simulink model "Model"  (R2015a)
settings: Solver=ode45  StartTime=0.0  StopTime=10.0  RelTol=1e-3
values from neighbouring files (symbols this model uses):
  A = [0          1          0           0 ... (first row only)    [ss_model.m]
  B = [0; 1; 0; 0]    [ss_model.m]
  C = [1 0 0 0 ... (first row only)    [ss_model.m]
  ctrl = 500/s    [ss_model.m]
  D = zeros(2,1)    [ss_model.m]
  Ke = -1.0000e+05    (= -100000)    [ss_model.m]    (also in synthesis.m)
  L = 0.0220    (= 0.022)    [ss_model.m]    (also in synthesis.m)
  R = 1.3    [ss_model.m]    (also in synthesis.m)
settings Model: CovModelRefEnable=off  Creator=gsavaia  LastModifiedBy=user
settings DataIOCC: SaveFormat=Dataset
settings HardwareCC: ProdBitPerPointer=64  ProdLargestAtomicFloat=Float  ProdIntDivRoundTo=Zero  ProdEndianess=LittleEndian  ProdHWDeviceType=Specified
settings GRTTargetCC: GeneratePreprocessorConditionals=Use local settings

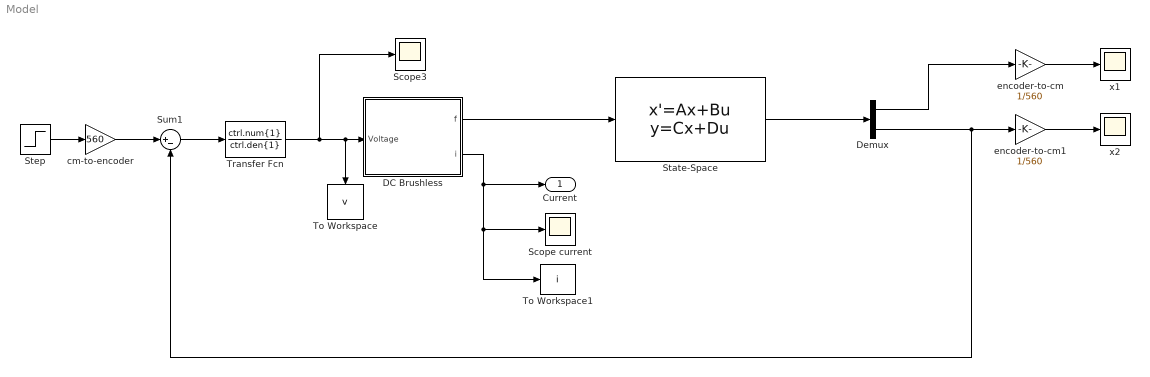
== system Model ==
  DC Brushless : Subsystem
  Demux : Demux  Outputs=2
  Scope current : Scope
      settings: YMin=-0.525  YMax=4.725
  Scope3 : Scope
      settings: TimeRange=2.475095785440614  YMin=3885000.000000001  YMax=8411666.666666668  SaveName=ScopeData4
  State-Space : StateSpace  A=A  B=B  C=C  D=D  X0=0
  Step : Step  SampleTime=0
  Sum1 : Sum  Inputs=|+-
  To Workspace : ToWorkspace  VariableName=v  SaveFormat=Timeseries  SampleTime=-1
  To Workspace1 : ToWorkspace  VariableName=i  SaveFormat=Timeseries  SampleTime=-1
  Transfer Fcn : TransferFcn  Numerator=ctrl.num{1}  Denominator=ctrl.den{1}
  cm-to-encoder : Gain  Gain=560
  encoder-to-cm : Gain  Gain=1/560
  encoder-to-cm1 : Gain  Gain=1/560
  x1 : Scope
      settings: YMin=-0.25393  YMax=2.28535
  x2 : Scope
      settings: TimeRange=10  YMin=-10  YMax=15  SaveName=ScopeData2
  Current : Outport
  wires:
  DC Brushless/1("f ") -> State-Space/1
  Transfer Fcn/1 -> To Workspace/1, DC Brushless/1("Voltage "), Scope3/1
  DC Brushless/2(i) -> Current/1, To Workspace1/1, Scope current/1
  Sum1/1 -> Transfer Fcn/1
  cm-to-encoder/1 -> Sum1/1
  Step/1 -> cm-to-encoder/1
  encoder-to-cm/1 -> x1/1
  State-Space/1 -> Demux/1
  Demux/1 -> encoder-to-cm/1
  encoder-to-cm1/1 -> x2/1
  Demux/2 -> Sum1/2, encoder-to-cm1/1

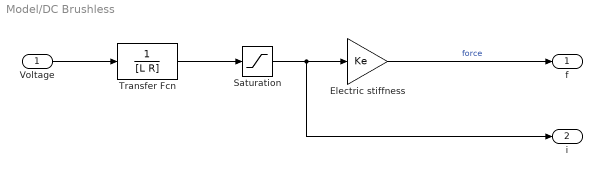
== system Model/DC Brushless ==
  "Voltage " : Inport
  Electric stiffness : Gain  Gain=Ke
  Saturation : Saturate  UpperLimit=4.2  LowerLimit=-10
  Transfer Fcn : TransferFcn  Denominator=[L R]
  "f " : Outport
  i : Outport  Port=2
  wires:
  "Voltage "/1 -> Transfer Fcn/1
  Electric stiffness/1 -> "f "/1  "force"
  Transfer Fcn/1 -> Saturation/1
  Saturation/1 -> i/1, Electric stiffness/1
